simulink model "ProcessModel_Boeing1"  (Simulink 7.9)
settings: Solver=VariableStepDiscrete  StartTime=0.0  StopTime=inf  RelTol=1e-3
libraries: simulink x1, simeventslib x1
settings Model: Creator=tsprock3  LastModifiedBy=tsprock3
settings DebuggingCC: UnconnectedInputMsg=none  UnconnectedOutputMsg=none  SimStateOlderReleaseMsg=warning

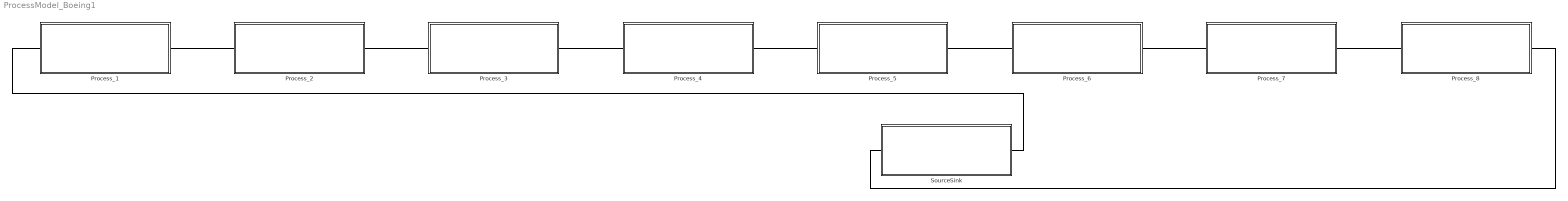
== system ProcessModel_Boeing1 ==
  Process_1 : Subsystem
  Process_2 : Subsystem
  Process_3 : Subsystem
  Process_4 : Subsystem
  Process_5 : Subsystem
  Process_6 : Subsystem
  Process_7 : Subsystem
  Process_8 : Subsystem
  SourceSink : Subsystem
  connections:
  Process_1/RConn1 -- Process_2/LConn1
  Process_2/RConn1 -- Process_3/LConn1
  Process_3/RConn1 -- Process_4/LConn1
  Process_4/RConn1 -- Process_5/LConn1
  Process_5/RConn1 -- Process_6/LConn1
  Process_6/RConn1 -- Process_7/LConn1
  Process_7/RConn1 -- Process_8/LConn1
  SourceSink/RConn1 -- Process_1/LConn1
  Process_8/RConn1 -- SourceSink/LConn1

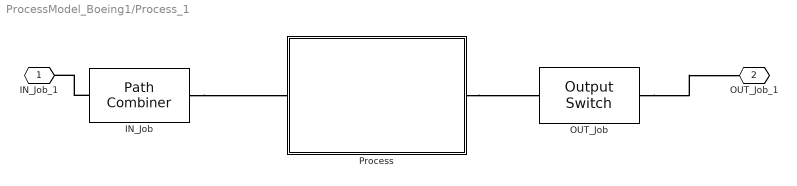
== system ProcessModel_Boeing1/Process_1 ==
  IN_Job : PathCombiner  NumberInputPorts=1
  OUT_Job : OutputSwitch  NumberOutputPorts=1
  Process : Subsystem
  IN_Job_1 : PMIOPort  Port=1  Side=Left
  OUT_Job_1 : PMIOPort  Port=2  Side=Right
  connections:
  Process/RConn1 -- OUT_Job/LConn1
  IN_Job/RConn1 -- Process/LConn1
  IN_Job/LConn1 -- IN_Job_1/RConn1
  OUT_Job/RConn1 -- OUT_Job_1/RConn1

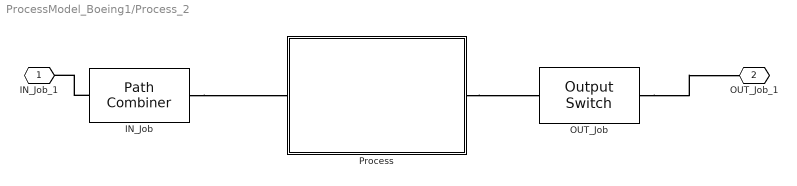
== system ProcessModel_Boeing1/Process_2 ==
  IN_Job : PathCombiner  NumberInputPorts=1
  OUT_Job : OutputSwitch  NumberOutputPorts=1
  Process : Subsystem
  IN_Job_1 : PMIOPort  Port=1  Side=Left
  OUT_Job_1 : PMIOPort  Port=2  Side=Right
  connections:
  Process/RConn1 -- OUT_Job/LConn1
  IN_Job/RConn1 -- Process/LConn1
  IN_Job/LConn1 -- IN_Job_1/RConn1
  OUT_Job/RConn1 -- OUT_Job_1/RConn1

== system ProcessModel_Boeing1/Process_3 ==
  IN_Job : PathCombiner  NumberInputPorts=1
  OUT_Job : OutputSwitch  NumberOutputPorts=1
  Process : Subsystem
  IN_Job_1 : PMIOPort  Port=1  Side=Left
  OUT_Job_1 : PMIOPort  Port=2  Side=Right
  connections:
  Process/RConn1 -- OUT_Job/LConn1
  IN_Job/RConn1 -- Process/LConn1
  IN_Job/LConn1 -- IN_Job_1/RConn1
  OUT_Job/RConn1 -- OUT_Job_1/RConn1

== system ProcessModel_Boeing1/Process_4 ==
  IN_Job : PathCombiner  NumberInputPorts=1
  OUT_Job : OutputSwitch  NumberOutputPorts=1
  Process : Subsystem
  IN_Job_1 : PMIOPort  Port=1  Side=Left
  OUT_Job_1 : PMIOPort  Port=2  Side=Right
  connections:
  Process/RConn1 -- OUT_Job/LConn1
  IN_Job/RConn1 -- Process/LConn1
  IN_Job/LConn1 -- IN_Job_1/RConn1
  OUT_Job/RConn1 -- OUT_Job_1/RConn1

== system ProcessModel_Boeing1/Process_5 ==
  IN_Job : PathCombiner  NumberInputPorts=1
  OUT_Job : OutputSwitch  NumberOutputPorts=1
  Process : Subsystem
  IN_Job_1 : PMIOPort  Port=1  Side=Left
  OUT_Job_1 : PMIOPort  Port=2  Side=Right
  connections:
  Process/RConn1 -- OUT_Job/LConn1
  IN_Job/RConn1 -- Process/LConn1
  IN_Job/LConn1 -- IN_Job_1/RConn1
  OUT_Job/RConn1 -- OUT_Job_1/RConn1

== system ProcessModel_Boeing1/Process_6 ==
  IN_Job : PathCombiner  NumberInputPorts=1
  OUT_Job : OutputSwitch  NumberOutputPorts=1
  Process : Subsystem
  IN_Job_1 : PMIOPort  Port=1  Side=Left
  OUT_Job_1 : PMIOPort  Port=2  Side=Right
  connections:
  Process/RConn1 -- OUT_Job/LConn1
  IN_Job/RConn1 -- Process/LConn1
  IN_Job/LConn1 -- IN_Job_1/RConn1
  OUT_Job/RConn1 -- OUT_Job_1/RConn1

== system ProcessModel_Boeing1/Process_7 ==
  IN_Job : PathCombiner  NumberInputPorts=1
  OUT_Job : OutputSwitch  NumberOutputPorts=1
  Process : Subsystem
  IN_Job_1 : PMIOPort  Port=1  Side=Left
  OUT_Job_1 : PMIOPort  Port=2  Side=Right
  connections:
  Process/RConn1 -- OUT_Job/LConn1
  IN_Job/RConn1 -- Process/LConn1
  IN_Job/LConn1 -- IN_Job_1/RConn1
  OUT_Job/RConn1 -- OUT_Job_1/RConn1

== system ProcessModel_Boeing1/Process_8 ==
  IN_Job : PathCombiner  NumberInputPorts=1
  OUT_Job : OutputSwitch  NumberOutputPorts=1
  Process : Subsystem
  IN_Job_1 : PMIOPort  Port=1  Side=Left
  OUT_Job_1 : PMIOPort  Port=2  Side=Right
  connections:
  Process/RConn1 -- OUT_Job/LConn1
  IN_Job/RConn1 -- Process/LConn1
  IN_Job/LConn1 -- IN_Job_1/RConn1
  OUT_Job/RConn1 -- OUT_Job_1/RConn1

== system ProcessModel_Boeing1/SourceSink ==
  IN_Job : EntityCombiner  NumberInputPorts=1  RetainComponentEntities=off
  OUT_Job : Replicate  NumberOutputPorts=1
  Process : Subsystem
  IN_Job_1 : PMIOPort  Port=1  Side=Left
  OUT_Job_1 : PMIOPort  Port=2  Side=Right
  connections:
  Process/RConn1 -- OUT_Job/LConn1
  IN_Job/RConn1 -- Process/LConn1
  IN_Job/LConn1 -- IN_Job_1/RConn1
  OUT_Job/RConn1 -- OUT_Job_1/RConn1

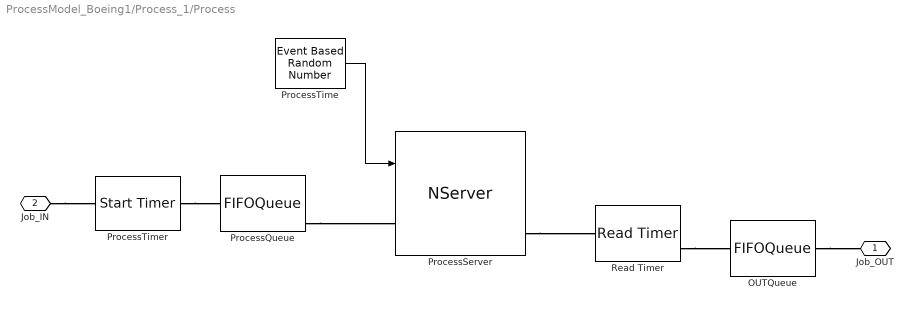
== system ProcessModel_Boeing1/Process_1/Process ==
  OUTQueue : FIFOQueue  Capacity=inf
  ProcessQueue : FIFOQueue  StatAverageWait=on  StatAverageQueueLength=on
      settings: OutputPortMap=o2,o3
  ProcessServer : NServer  NumberOfServers=1  ServiceTimeFrom=Signal port t  StatNumberDeparted=on  StatUtilization=on
      settings: OutputPortMap=o0,o5
  ProcessTime : EventBasedRandomNumber  Distribution=Gaussian (normal)  minUnif=1  meanNorm=3  stdNorm=0.3  Seed=4276
  ProcessTimer : StartTimer  TimerTag=T_Process_1  TimerStartedOption=Restart
  Read Timer : ReadTimer  TimerTag=T_Process_1  StatAverageTimeElapsed=on
      settings: OutputPortMap=o3
  Job_OUT : PMIOPort  Port=1  Side=Right
  Job_IN : PMIOPort  Port=2  Side=Left
  wires:
  ProcessTime/1 -> ProcessServer/1
  connections:
  OUTQueue/RConn1 -- Job_OUT/RConn1
  Read Timer/RConn1 -- OUTQueue/LConn1
  ProcessQueue/RConn1 -- ProcessServer/LConn1
  ProcessTimer/RConn1 -- ProcessQueue/LConn1
  ProcessServer/RConn1 -- Read Timer/LConn1
  Job_IN/RConn1 -- ProcessTimer/LConn1

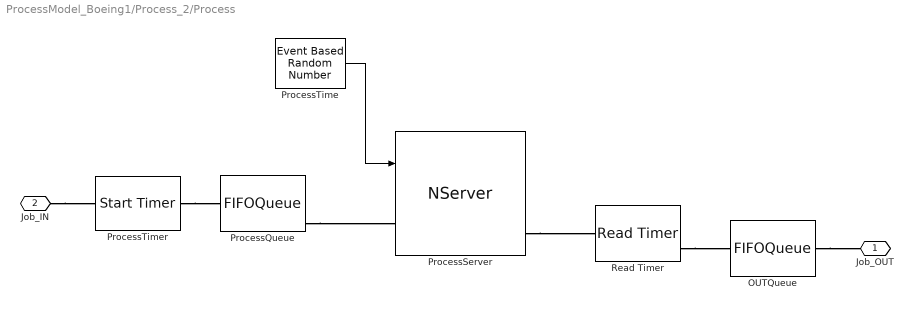
== system ProcessModel_Boeing1/Process_2/Process ==
  OUTQueue : FIFOQueue  Capacity=inf
  ProcessQueue : FIFOQueue  StatAverageWait=on  StatAverageQueueLength=on
      settings: OutputPortMap=o2,o3
  ProcessServer : NServer  NumberOfServers=1  ServiceTimeFrom=Signal port t  StatNumberDeparted=on  StatUtilization=on
      settings: OutputPortMap=o0,o5
  ProcessTime : EventBasedRandomNumber  Distribution=Gaussian (normal)  minUnif=1  meanNorm=2  stdNorm=0.2  Seed=4276
  ProcessTimer : StartTimer  TimerTag=T_Process_2  TimerStartedOption=Restart
  Read Timer : ReadTimer  TimerTag=T_Process_2  StatAverageTimeElapsed=on
      settings: OutputPortMap=o3
  Job_OUT : PMIOPort  Port=1  Side=Right
  Job_IN : PMIOPort  Port=2  Side=Left
  wires:
  ProcessTime/1 -> ProcessServer/1
  connections:
  OUTQueue/RConn1 -- Job_OUT/RConn1
  Read Timer/RConn1 -- OUTQueue/LConn1
  ProcessQueue/RConn1 -- ProcessServer/LConn1
  ProcessTimer/RConn1 -- ProcessQueue/LConn1
  ProcessServer/RConn1 -- Read Timer/LConn1
  Job_IN/RConn1 -- ProcessTimer/LConn1

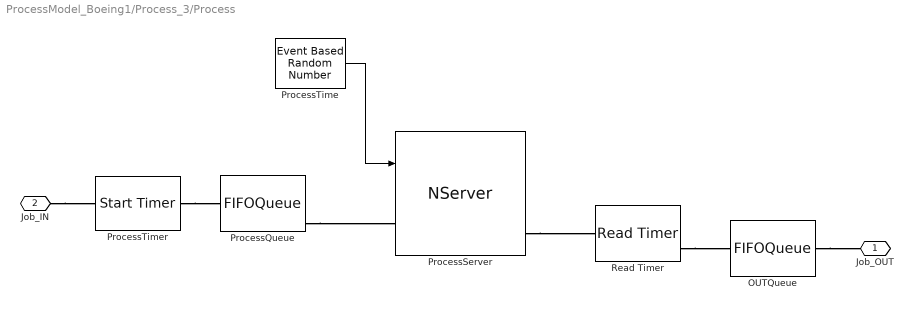
== system ProcessModel_Boeing1/Process_3/Process ==
  OUTQueue : FIFOQueue  Capacity=inf
  ProcessQueue : FIFOQueue  StatAverageWait=on  StatAverageQueueLength=on
      settings: OutputPortMap=o2,o3
  ProcessServer : NServer  NumberOfServers=1  ServiceTimeFrom=Signal port t  StatNumberDeparted=on  StatUtilization=on
      settings: OutputPortMap=o0,o5
  ProcessTime : EventBasedRandomNumber  Distribution=Gaussian (normal)  minUnif=1  meanNorm=1  stdNorm=0.1  Seed=4276
  ProcessTimer : StartTimer  TimerTag=T_Process_3  TimerStartedOption=Restart
  Read Timer : ReadTimer  TimerTag=T_Process_3  StatAverageTimeElapsed=on
      settings: OutputPortMap=o3
  Job_OUT : PMIOPort  Port=1  Side=Right
  Job_IN : PMIOPort  Port=2  Side=Left
  wires:
  ProcessTime/1 -> ProcessServer/1
  connections:
  OUTQueue/RConn1 -- Job_OUT/RConn1
  Read Timer/RConn1 -- OUTQueue/LConn1
  ProcessQueue/RConn1 -- ProcessServer/LConn1
  ProcessTimer/RConn1 -- ProcessQueue/LConn1
  ProcessServer/RConn1 -- Read Timer/LConn1
  Job_IN/RConn1 -- ProcessTimer/LConn1

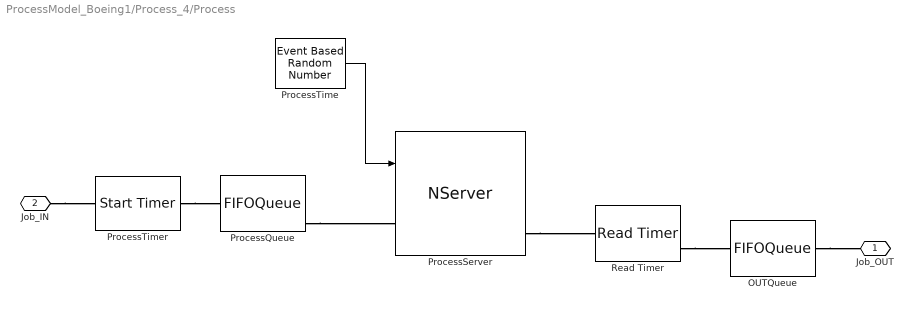
== system ProcessModel_Boeing1/Process_4/Process ==
  OUTQueue : FIFOQueue  Capacity=inf
  ProcessQueue : FIFOQueue  StatAverageWait=on  StatAverageQueueLength=on
      settings: OutputPortMap=o2,o3
  ProcessServer : NServer  NumberOfServers=1  ServiceTimeFrom=Signal port t  StatNumberDeparted=on  StatUtilization=on
      settings: OutputPortMap=o0,o5
  ProcessTime : EventBasedRandomNumber  Distribution=Gaussian (normal)  minUnif=1  meanNorm=2  stdNorm=0.2  Seed=4276
  ProcessTimer : StartTimer  TimerTag=T_Process_4  TimerStartedOption=Restart
  Read Timer : ReadTimer  TimerTag=T_Process_4  StatAverageTimeElapsed=on
      settings: OutputPortMap=o3
  Job_OUT : PMIOPort  Port=1  Side=Right
  Job_IN : PMIOPort  Port=2  Side=Left
  wires:
  ProcessTime/1 -> ProcessServer/1
  connections:
  OUTQueue/RConn1 -- Job_OUT/RConn1
  Read Timer/RConn1 -- OUTQueue/LConn1
  ProcessQueue/RConn1 -- ProcessServer/LConn1
  ProcessTimer/RConn1 -- ProcessQueue/LConn1
  ProcessServer/RConn1 -- Read Timer/LConn1
  Job_IN/RConn1 -- ProcessTimer/LConn1

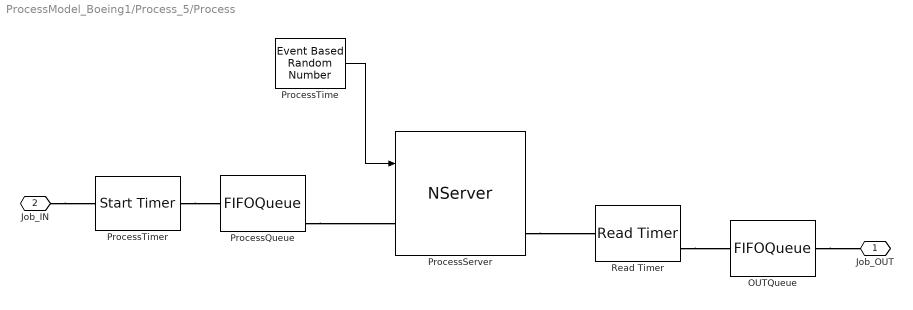
== system ProcessModel_Boeing1/Process_5/Process ==
  OUTQueue : FIFOQueue  Capacity=inf
  ProcessQueue : FIFOQueue  StatAverageWait=on  StatAverageQueueLength=on
      settings: OutputPortMap=o2,o3
  ProcessServer : NServer  NumberOfServers=1  ServiceTimeFrom=Signal port t  StatNumberDeparted=on  StatUtilization=on
      settings: OutputPortMap=o0,o5
  ProcessTime : EventBasedRandomNumber  Distribution=Gaussian (normal)  minUnif=1  meanNorm=1  stdNorm=0.1  Seed=4276
  ProcessTimer : StartTimer  TimerTag=T_Process_5  TimerStartedOption=Restart
  Read Timer : ReadTimer  TimerTag=T_Process_5  StatAverageTimeElapsed=on
      settings: OutputPortMap=o3
  Job_OUT : PMIOPort  Port=1  Side=Right
  Job_IN : PMIOPort  Port=2  Side=Left
  wires:
  ProcessTime/1 -> ProcessServer/1
  connections:
  OUTQueue/RConn1 -- Job_OUT/RConn1
  Read Timer/RConn1 -- OUTQueue/LConn1
  ProcessQueue/RConn1 -- ProcessServer/LConn1
  ProcessTimer/RConn1 -- ProcessQueue/LConn1
  ProcessServer/RConn1 -- Read Timer/LConn1
  Job_IN/RConn1 -- ProcessTimer/LConn1

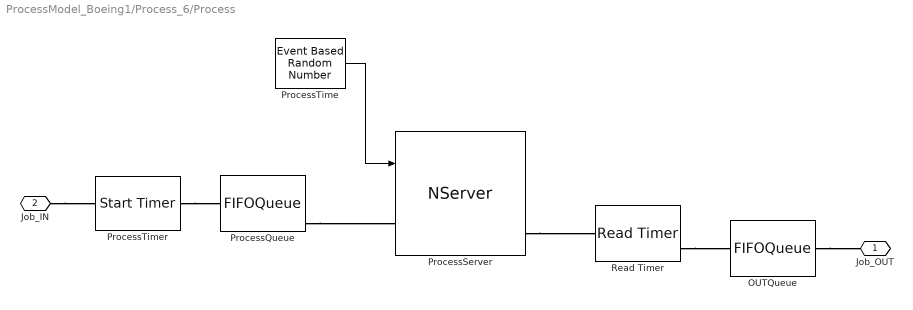
== system ProcessModel_Boeing1/Process_6/Process ==
  OUTQueue : FIFOQueue  Capacity=inf
  ProcessQueue : FIFOQueue  StatAverageWait=on  StatAverageQueueLength=on
      settings: OutputPortMap=o2,o3
  ProcessServer : NServer  NumberOfServers=1  ServiceTimeFrom=Signal port t  StatNumberDeparted=on  StatUtilization=on
      settings: OutputPortMap=o0,o5
  ProcessTime : EventBasedRandomNumber  Distribution=Gaussian (normal)  minUnif=1  meanNorm=2  stdNorm=0.2  Seed=4276
  ProcessTimer : StartTimer  TimerTag=T_Process_6  TimerStartedOption=Restart
  Read Timer : ReadTimer  TimerTag=T_Process_6  StatAverageTimeElapsed=on
      settings: OutputPortMap=o3
  Job_OUT : PMIOPort  Port=1  Side=Right
  Job_IN : PMIOPort  Port=2  Side=Left
  wires:
  ProcessTime/1 -> ProcessServer/1
  connections:
  OUTQueue/RConn1 -- Job_OUT/RConn1
  Read Timer/RConn1 -- OUTQueue/LConn1
  ProcessQueue/RConn1 -- ProcessServer/LConn1
  ProcessTimer/RConn1 -- ProcessQueue/LConn1
  ProcessServer/RConn1 -- Read Timer/LConn1
  Job_IN/RConn1 -- ProcessTimer/LConn1

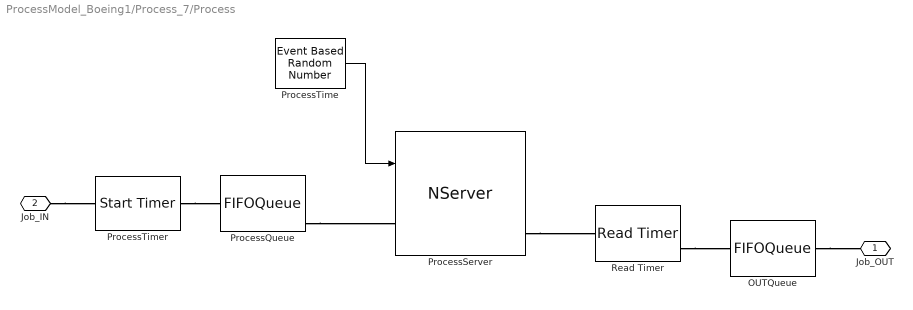
== system ProcessModel_Boeing1/Process_7/Process ==
  OUTQueue : FIFOQueue  Capacity=inf
  ProcessQueue : FIFOQueue  StatAverageWait=on  StatAverageQueueLength=on
      settings: OutputPortMap=o2,o3
  ProcessServer : NServer  NumberOfServers=1  ServiceTimeFrom=Signal port t  StatNumberDeparted=on  StatUtilization=on
      settings: OutputPortMap=o0,o5
  ProcessTime : EventBasedRandomNumber  Distribution=Gaussian (normal)  minUnif=1  meanNorm=4  stdNorm=0.4  Seed=4276
  ProcessTimer : StartTimer  TimerTag=T_Process_7  TimerStartedOption=Restart
  Read Timer : ReadTimer  TimerTag=T_Process_7  StatAverageTimeElapsed=on
      settings: OutputPortMap=o3
  Job_OUT : PMIOPort  Port=1  Side=Right
  Job_IN : PMIOPort  Port=2  Side=Left
  wires:
  ProcessTime/1 -> ProcessServer/1
  connections:
  OUTQueue/RConn1 -- Job_OUT/RConn1
  Read Timer/RConn1 -- OUTQueue/LConn1
  ProcessQueue/RConn1 -- ProcessServer/LConn1
  ProcessTimer/RConn1 -- ProcessQueue/LConn1
  ProcessServer/RConn1 -- Read Timer/LConn1
  Job_IN/RConn1 -- ProcessTimer/LConn1

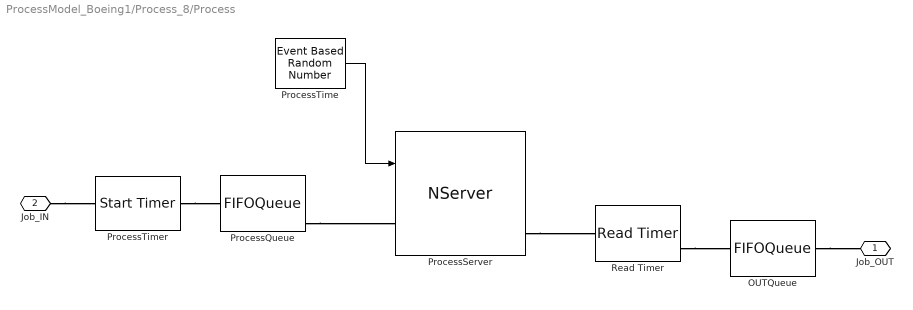
== system ProcessModel_Boeing1/Process_8/Process ==
  OUTQueue : FIFOQueue  Capacity=inf
  ProcessQueue : FIFOQueue  StatAverageWait=on  StatAverageQueueLength=on
      settings: OutputPortMap=o2,o3
  ProcessServer : NServer  NumberOfServers=1  ServiceTimeFrom=Signal port t  StatNumberDeparted=on  StatUtilization=on
      settings: OutputPortMap=o0,o5
  ProcessTime : EventBasedRandomNumber  Distribution=Gaussian (normal)  minUnif=1  meanNorm=3  stdNorm=0.3  Seed=4276
  ProcessTimer : StartTimer  TimerTag=T_Process_8  TimerStartedOption=Restart
  Read Timer : ReadTimer  TimerTag=T_Process_8  StatAverageTimeElapsed=on
      settings: OutputPortMap=o3
  Job_OUT : PMIOPort  Port=1  Side=Right
  Job_IN : PMIOPort  Port=2  Side=Left
  wires:
  ProcessTime/1 -> ProcessServer/1
  connections:
  OUTQueue/RConn1 -- Job_OUT/RConn1
  Read Timer/RConn1 -- OUTQueue/LConn1
  ProcessQueue/RConn1 -- ProcessServer/LConn1
  ProcessTimer/RConn1 -- ProcessQueue/LConn1
  ProcessServer/RConn1 -- Read Timer/LConn1
  Job_IN/RConn1 -- ProcessTimer/LConn1

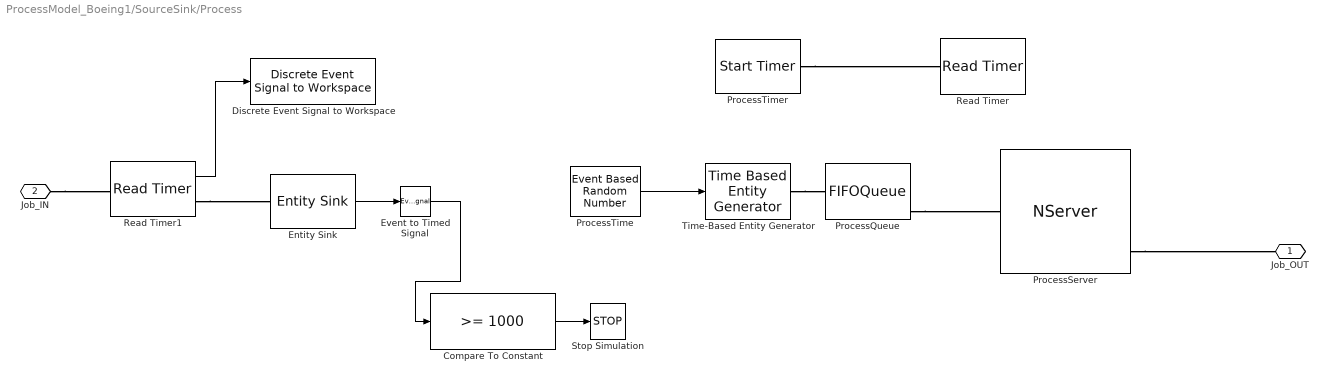
== system ProcessModel_Boeing1/SourceSink/Process ==
  Compare To Constant : simulink/Logic and Bit Operations/Compare To Constant  relop=>=  const=1000  OutDataTypeStr=boolean
  Discrete Event Signal to Workspace : simeventslib/SimEvents Sinks/Discrete Event Signal to Workspace  VariableName=ProcessTime  SaveFormat=Structure With Time  isMonitorOnly=off  isRecordIC=off
  Entity Sink : EntitySink  StatNumberArrived=on
  Event to Timed Signal : EventToTimedSignal
  ProcessQueue : FIFOQueue  StatAverageWait=on  StatAverageQueueLength=on
      settings: OutputPortMap=o2,o3
  ProcessServer : NServer  NumberOfServers=1  ServiceTime=0  StatNumberDeparted=on  StatUtilization=on
      settings: OutputPortMap=o0,o5
  ProcessTime : EventBasedRandomNumber  Distribution=Gaussian (normal)  minUnif=1  meanNorm=1  stdNorm=0.001  Seed=4276
  ProcessTimer : StartTimer  TimerTag=T_SourceSink  TimerStartedOption=Restart
  Read Timer : ReadTimer  TimerTag=T_SourceSink  StatAverageTimeElapsed=on
      settings: OutputPortMap=o3
  Read Timer1 : ReadTimer  TimerTag=T_Process_1  StatTimeElapsed=on
      settings: OutputPortMap=o2
  Stop Simulation : Stop
  Time-Based Entity Generator : TimeBasedEntityGenerator  GenerateEntitiesUpon=Intergeneration time from port t
  Job_OUT : PMIOPort  Port=1  Side=Right
  Job_IN : PMIOPort  Port=2  Side=Left
  wires:
  Entity Sink/1 -> Event to Timed Signal/1
  Event to Timed Signal/1 -> Compare To Constant/1
  Compare To Constant/1 -> Stop Simulation/1
  Read Timer1/1 -> Discrete Event Signal to Workspace/1
  ProcessTime/1 -> Time-Based Entity Generator/1
  connections:
  Job_IN/RConn1 -- Read Timer1/LConn1
  Read Timer1/RConn1 -- Entity Sink/LConn1
  ProcessServer/RConn1 -- Job_OUT/RConn1
  Time-Based Entity Generator/RConn1 -- ProcessQueue/LConn1
  ProcessTimer/RConn1 -- Read Timer/LConn1
  ProcessQueue/RConn1 -- ProcessServer/LConn1
